simulink model "ssb2"  (R2021b)
settings: Solver=ode45  StartTime=0.0  StopTime=0.001  RelTol=1e-3
libraries: dsparch4 x1
settings Model: Creator=Dell  LastModifiedBy=Dell
settings SolverCC: AlgebraicLoopSolver=TrustRegion
settings DataIOCC: LimitDataPoints=on  SaveOutput=off  SaveTime=off
settings OptimizationCC: BooleanDataType=off  DefaultParameterBehavior=Inlined  LocalBlockOutputs=off  LifeSpan=inf
settings DebuggingCC: AlgebraicLoopMsg=error  SingleTaskRateTransMsg=error  AllowSymbolicDim=off  SFUnexpectedBacktrackingDiag=warning  SFNoUnconditionalDefaultTransitionDiag=warning  SFExecutionAtInitializationDiag=none  SFMachineParentedDataDiag=warning  ArithmeticOperatorsInVariantConditions=warning
settings SFSimCC: SimUseLocalCustomCode=off  CustomCodeUndefinedFunction=UseInterfaceOnly
settings RTWCC: RTWUseLocalCustomCode=off
settings CodeAppCC: StateflowObjectComments=on
settings GRTTargetCC: TargetLangStandard=C89/C90 (ANSI)
settings ConfigComp: CovMetricSettings=dw  CovSaveCumulativeToWorkspaceVar=on  CovSaveSingleToWorkspaceVar=on  CovExternalEMLEnable=off  CovSFcnEnable=off

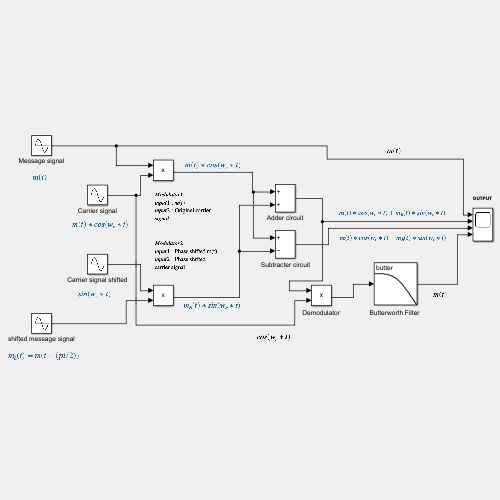
[thumbnail: Simulink's stored preview of the top-level diagram]
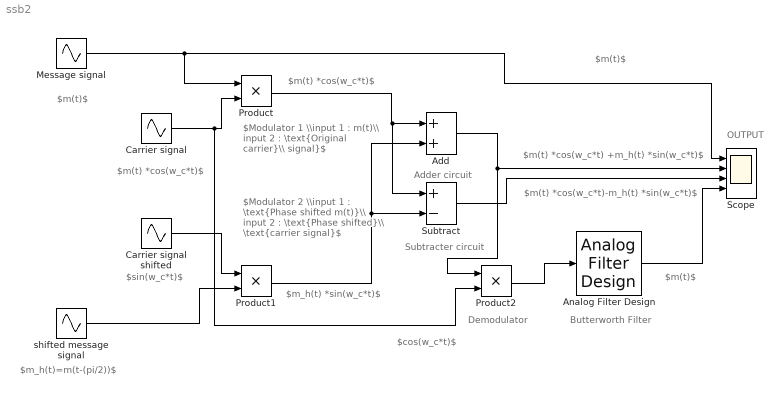
== system ssb2 ==
  note: OUTPUT
  note: $m(t) *cos(w_c*t) +m_h(t) *sin(w_c*t)$
  note: Butterworth Filter
  note: Demodulator
  note: Adder circuit
  note: $Modulator 1 \\input 1 : m(t)\\ input 2 : \text{Original carrier}\\ signal}$
  note: $sin(w_c*t)$
  note: $m(t) *cos(w_c*t)$
  note: $m_h(t)=m(t-(pi/2))$
  note: $m(t)$
  note: $Modulator 2 \\input 1 : \text{Phase shifted m(t)}\\ input 2 : \text{Phase shifted}\\ \text{carrier signal}$
  note: $m_h(t) *sin(w_c*t)$
  note: $m(t) *cos(w_c*t)$
  note: $cos(w_c*t)$
  note: $m(t)$
  note: $m(t)$
  note: Subtracter circuit
  note: $m(t) *cos(w_c*t)-m_h(t) *sin(w_c*t)$
  Add : Sum
  Analog Filter Design : dsparch4/Analog Filter Design  method=Butterworth  filttype=Lowpass  N=1  Wlo=2*pi*2000  Whi=80  Rp=2  Rs=40
  Carrier signal : Sin  Frequency=2*pi*100000  Phase=-(pi/2)  SampleTime=0
  Carrier signal shifted : Sin  Frequency=2*pi*100000  SampleTime=0
  Message signal : Sin  Frequency=2*pi*2000  SampleTime=0
  Product : Product
  Product1 : Product
  Product2 : Product
  Scope : Scope  NumInputPorts=4
  Subtract : Sum  Inputs=+-
  shifted message signal : Sin  Frequency=2*pi*2000  Phase=-(pi/2)  SampleTime=0
  wires:
  Carrier signal/1 -> Product/2, Product2/2
  Carrier signal shifted/1 -> Product1/1
  Product1/1 -> Subtract/2, Add/2
  Product/1 -> Subtract/1, Add/1
  Add/1 -> Product2/1, Scope/2
  Product2/1 -> Analog Filter Design/1
  Analog Filter Design/1 -> Scope/4
  Message signal/1 -> Product/1, Scope/1
  shifted message signal/1 -> Product1/2
  Subtract/1 -> Scope/3
